simulink model "stm32g474_buck_vmc_discoverykit"  (R2022a)
settings: Solver=FixedStepAuto  StartTime=0.0  StopTime=inf  RelTol=1e-3  EnableMultiTasking=on
libraries: stm32f4xxblockslib x5, stm32g4xxblockslib x3, simulink x2, stm32blockslib x1, svdutilitieslib x1
settings Model: Creator=vchilapu  LastModifiedBy=User
settings SolverCC: MaxZcPerStep=1
settings OptimizationCC: DefaultUnderspecifiedDataType=single  EnhancedBackFolding=on  PassReuseOutputArgsAs=Individual arguments  ZeroExternalMemoryAtStartup=off  ZeroInternalMemoryAtStartup=off  MaxStackSize=64  OptimizeBlockOrder=speed  DifferentSizesBufferReuse=on  OptimizationCustomize=off  EfficientTunableParamExpr=on
settings DebuggingCC: ParameterPrecisionLossMsg=none  ParameterTunabilityLossMsg=error
settings HardwareCC: ProdBitPerPointer=32  ProdBitPerSizeT=32  ProdBitPerPtrDiffT=32  ProdLargestAtomicInteger=Long  ProdLargestAtomicFloat=Double  ProdWordSize=32  ProdLongLongMode=on  ProdHWDeviceType=ARM Compatible->ARM Cortex
settings SFSimCC: MATLABDynamicMemAlloc=off
settings RTWCC: SystemTargetFile=ert.tlc  HardwareBoard=STM32G4xx Based  TemplateMakefile=ert_default_tmf  GenerateReport=on  Toolchain=GNU Tools for ARM Embedded Processors  BuildConfiguration=Specify  IncludeHyperlinkInReport=on  GenerateTraceInfo=on
settings CodeAppCC: ForceParamTrailComments=on  IgnoreCustomStorageClasses=off  OperatorAnnotations=on  SimulinkDataObjDesc=on  SFDataObjDesc=on  InsertBlockDesc=on
settings ERTTargetCC: TargetLangStandard=C99 (ISO)  CodeReplacementLibrary=ARM Cortex-M  ExtModeTransport=3  ExtModeStaticAlloc=on  ExtModeStaticAllocSize=2048  ExtModeMexFile=ext_xcp  ExtModeIntrfLevel=Level2 - Open

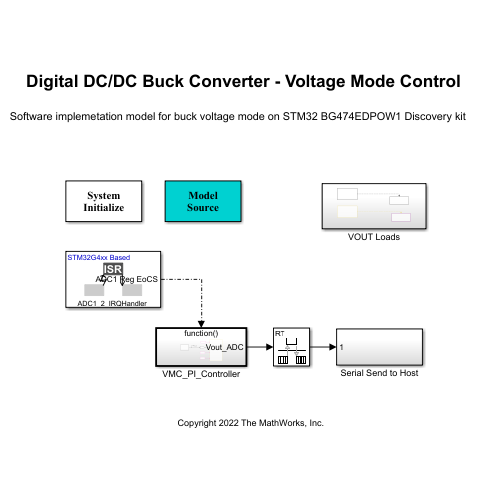
[thumbnail: Simulink's stored preview of the top-level diagram]
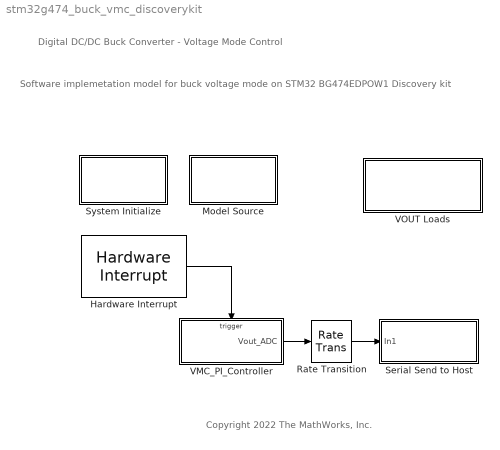
== system stm32g474_buck_vmc_discoverykit ==
  note: Digital DC/DC Buck Converter - Voltage Mode Control
  note: Software implemetation model for buck voltage mode on STM32 BG474EDPOW1 Discovery kit
  note: Copyright 2022 The MathWorks, Inc.
  Hardware Interrupt : stm32g4xxblockslib/Hardware Interrupt  ISRGroup=Analog to digital converter (ADC)  ISRName=ADC1_2_IRQHandler  ISRNumber=33  EventsList={ 'off', 'ADC1 OVR', '1'; 'on', 'ADC1 Reg EoCS', '2'; 'off', 'ADC1 Inj EoCS', '3'; 'off', 'ADC1 Inj JQOVF', '4'; 'off', 'ADC1 Watchdog1', '5'; 'off', 'ADC1 Watchdog2', '6'; 'off', 'ADC1 Watchdog3', '7'; 'off', 'ADC2 OVR', '8'; 'off', 'ADC2 Reg EoCS', '9'; 'off', 'ADC2 Inj EoCS', '10'; 'off', 'ADC2 Inj JQOVF', '11'; 'off', 'ADC2 Watchdog', '12'; 'off', 'ADC2 Watchdog2', '13'; 'off', 'ADC2 Watchdog3', '14'; 'off', 'Custom event', '15' }  SelectedEvents={'ADC1 Reg EoCS'}  TaskPriority=30  DisablePreemption=off  ClearInterruptFlagsAtEndOfEvent=off  InterruptDefinitionFile=$(TARGET_ROOT)/registry/interrupts/STM32F4xxBased_interrupts.xml  EnableSimPort=off
      settings: SourceProductBaseCode=STMICRODIS
  Model Source : Subsystem  mask(Model Source){ShowInLibBrowser=0}
      mask prompts: ShowInLibBrowser "Simulink:masks:CustCodeMaskParam1_MP"
      settings: CopyFcn=cccopyfcn(gcb)  OpenFcn=ccopenfcn('Model Source')
      mask Help: eval('feval(''rtwprivate'',''rtwhelpview'',''rtw_model_source_block'')');
      mask Display: disp('Model\nSource');
  Rate Transition : RateTransition  Integrity=off  Deterministic=off  OutPortSampleTime=20e-6
  Serial Send to Host : Subsystem
  System Initialize : Subsystem  mask(System Initialize){ShowInLibBrowser=0}
      mask prompts: ShowInLibBrowser "Simulink:masks:CustCodeMaskParam1_MP"
      settings: CopyFcn=cccopyfcn(gcb)  OpenFcn=ccopenfcn('System Initialize Function')
      mask Help: eval('feval(''rtwprivate'',''rtwhelpview'',''rtw_sys_initialize_block'')');
      mask Display: disp('System\nInitialize');
  VMC_PI_Controller : Subsystem  TreatAsAtomicUnit=on
  VOUT Loads : Subsystem
  wires:
  VMC_PI_Controller/1(Vout_ADC) -> Rate Transition/1
  Rate Transition/1 -> Serial Send to Host/1(In1)
  Hardware Interrupt/1 -> VMC_PI_Controller/Trigger

== system stm32g474_buck_vmc_discoverykit/Model Source ==

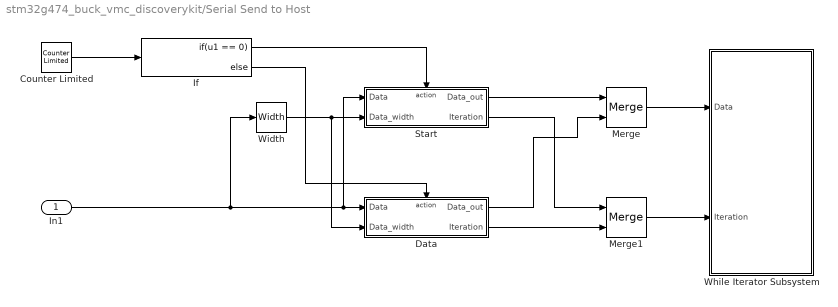
== system stm32g474_buck_vmc_discoverykit/Serial Send to Host ==
  In1 : Inport
  Counter Limited : simulink/Sources/Counter Limited  uplimit=2999  tsamp=-1
  Data : Subsystem  TreatAsAtomicUnit=on
  If : If  IfExpression=u1 == 0
  Merge : Merge
  Merge1 : Merge
  Start : Subsystem  TreatAsAtomicUnit=on
  While Iterator Subsystem : Subsystem  TreatAsAtomicUnit=on
  Width : Width  OutDataTypeMode=All ports same datatype  DataType=uint16
  wires:
  If/1 -> Start/Action
  If/2 -> Data/Action
  Counter Limited/1 -> If/1
  Start/1(Data_out) -> Merge/1
  Data/1(Data_out) -> Merge/2
  Merge/1 -> While Iterator Subsystem/1(Data)
  Merge1/1 -> While Iterator Subsystem/2(Iteration)
  Start/2(Iteration) -> Merge1/1
  Data/2(Iteration) -> Merge1/2
  Width/1 -> Data/2(Data_width), Start/2(Data_width)
  In1/1 -> Width/1, Start/1(Data), Data/1(Data)

== system stm32g474_buck_vmc_discoverykit/System Initialize ==

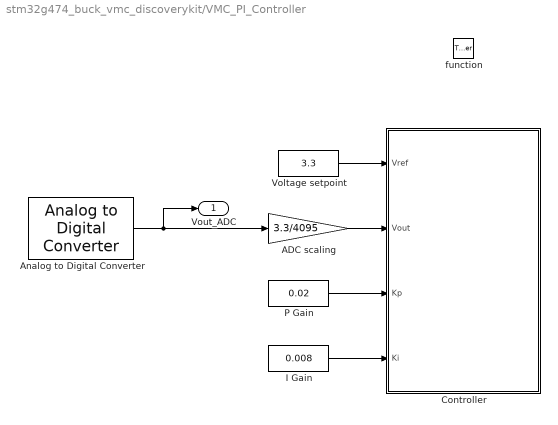
== system stm32g474_buck_vmc_discoverykit/VMC_PI_Controller ==
  function : TriggerPort  TriggerType=function-call  VariantControl=(inherit)
  ADC scaling : Gain  Gain=3.3/4095  OutDataTypeStr=single
  Analog to Digital Converter : stm32f4xxblockslib/Analog to Digital Converter  ADCModule=ADC1  ConversionGroup=Regular  TriggerMode=Read results only  NumberOfConversions=1  OutputStatus=off  SampleTime=-1  EnableSimPort=off
      settings: SourceProductBaseCode=STMICRODIS
  Controller : Subsystem
  I Gain : Constant  Value=0.008  VectorParams1D=off  OutDataTypeStr=Inherit: Inherit via back propagation
  P Gain : Constant  Value=0.02  OutDataTypeStr=Inherit: Inherit via back propagation
  Voltage setpoint : Constant  Value=3.3  OutDataTypeStr=Inherit: Inherit via back propagation
  Vout_ADC : Outport
  wires:
  ADC scaling/1 -> Controller/2(Vout)
  P Gain/1 -> Controller/3(Kp)
  I Gain/1 -> Controller/4(Ki)
  Analog to Digital Converter/1 -> Vout_ADC/1, ADC scaling/1
  Voltage setpoint/1 -> Controller/1(Vref)

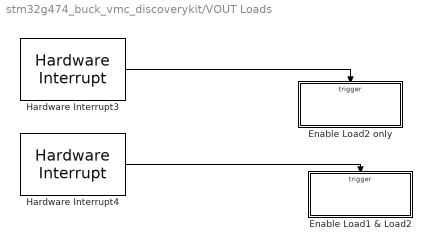
== system stm32g474_buck_vmc_discoverykit/VOUT Loads ==
  Enable Load1 & Load2 : Subsystem  TreatAsAtomicUnit=on
  Enable Load2 only : Subsystem  TreatAsAtomicUnit=on
  Hardware Interrupt3 : stm32g4xxblockslib/Hardware Interrupt  ISRGroup=External interrupts (EXTI)  ISRName=EXTI2_IRQHandler  ISRNumber=23  EventsList={ 'on', 'EXTI2 Event', '1'; 'off', 'Custom event', '2' }  SelectedEvents={'EXTI2 Event'}  TaskPriority=30  DisablePreemption=off  ClearInterruptFlagsAtEndOfEvent=off  InterruptDefinitionFile=$(TARGET_ROOT)/registry/interrupts/STM32F4xxBased_interrupts.xml  EnableSimPort=off
      settings: SourceProductBaseCode=STMICRODIS
  Hardware Interrupt4 : stm32g4xxblockslib/Hardware Interrupt  ISRGroup=External interrupts (EXTI)  ISRName=EXTI4_IRQHandler  ISRNumber=25  EventsList={ 'on', 'EXTI4 Event', '1'; 'off', 'Custom event', '2' }  SelectedEvents={'EXTI4 Event'}  TaskPriority=30  DisablePreemption=off  ClearInterruptFlagsAtEndOfEvent=off  InterruptDefinitionFile=$(TARGET_ROOT)/registry/interrupts/STM32F4xxBased_interrupts.xml  EnableSimPort=off
      settings: SourceProductBaseCode=STMICRODIS
  wires:
  Hardware Interrupt3/1 -> Enable Load2 only/Trigger
  Hardware Interrupt4/1 -> Enable Load1 & Load2/Trigger

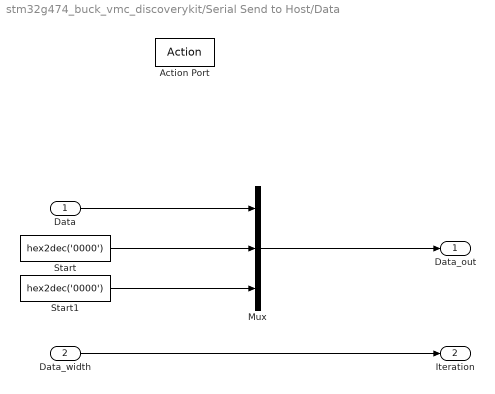
== system stm32g474_buck_vmc_discoverykit/Serial Send to Host/Data ==
  Data : Inport
  Data_width : Inport  Port=2
  Action Port : ActionPort  ActionPortLabel=else
  Mux : Mux  Inputs=3
  Start : Constant  Value=hex2dec('0000')  OutDataTypeStr=uint16
  Start1 : Constant  Value=hex2dec('0000')  OutDataTypeStr=uint16
  Data_out : Outport  VectorParamsAs1DForOutWhenUnconnected=off
  Iteration : Outport  Port=2  VectorParamsAs1DForOutWhenUnconnected=off
  wires:
  Start/1 -> Mux/2
  Mux/1 -> Data_out/1
  Data/1 -> Mux/1
  Data_width/1 -> Iteration/1
  Start1/1 -> Mux/3

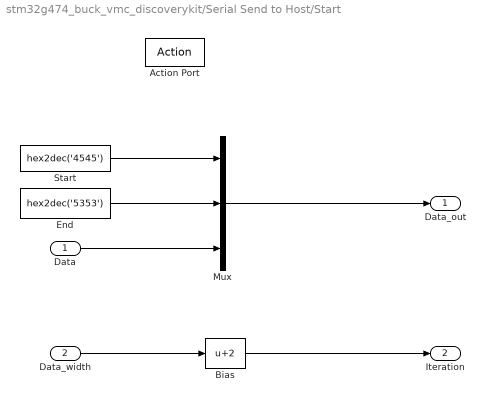
== system stm32g474_buck_vmc_discoverykit/Serial Send to Host/Start ==
  Data : Inport
  Data_width : Inport  Port=2
  Action Port : ActionPort  ActionPortLabel=if(u1 == 0)
  Bias : Bias  Bias=2  SaturateOnIntegerOverflow=off
  End : Constant  Value=hex2dec('5353')  OutDataTypeStr=uint16
  Mux : Mux  Inputs=3
  Start : Constant  Value=hex2dec('4545')  OutDataTypeStr=uint16
  Data_out : Outport  VectorParamsAs1DForOutWhenUnconnected=off
  Iteration : Outport  Port=2  VectorParamsAs1DForOutWhenUnconnected=off
  wires:
  End/1 -> Mux/2
  Mux/1 -> Data_out/1
  Data_width/1 -> Bias/1
  Bias/1 -> Iteration/1
  Data/1 -> Mux/3
  Start/1 -> Mux/1

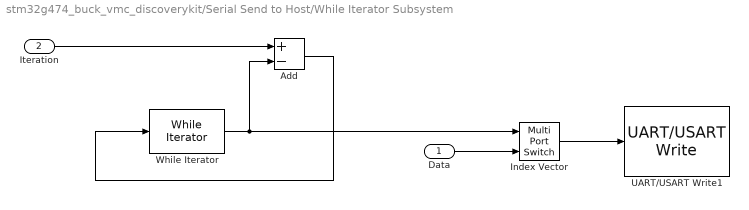
== system stm32g474_buck_vmc_discoverykit/Serial Send to Host/While Iterator Subsystem ==
  Data : Inport
  Iteration : Inport  Port=2
  Add : Sum  Inputs=+-  OutDataTypeStr=Inherit: Same as first input
  Index Vector : MultiPortSwitch  Inputs=1  SaturateOnIntegerOverflow=off  InputSameDT=off
  UART/USART Write1 : stm32blockslib/UART//USART Write  Priority=1  UARTModule=USART3  LengthOfDataToSend=off  BlockingMode=on  BlockingTimeout=1  OutputStatus=off
      settings: SourceProductBaseCode=STMICRODIS
  While Iterator : WhileIterator  MaxIters=-1  WhileBlockType=do-while  ShowIterationPort=on  OutputDataType=int16
  wires:
  Iteration/1 -> Add/1
  Add/1 -> While Iterator/1
  Index Vector/1 -> UART/USART Write1/1
  Data/1 -> Index Vector/2
  While Iterator/1 -> Index Vector/1, Add/2

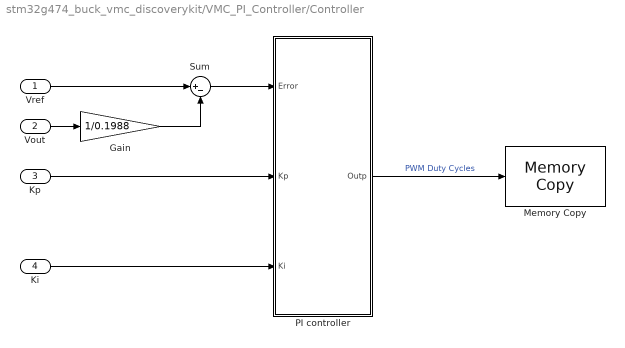
== system stm32g474_buck_vmc_discoverykit/VMC_PI_Controller/Controller ==
  Vref : Inport
  Vout : Inport  Port=2
  Kp : Inport  Port=3
  Ki : Inport  Port=4
  Gain : Gain  Gain=1/0.1988
  Memory Copy : svdutilitieslib/Memory Copy  copyFrom=Input port  copyFromAddressSource=Specify via dialog  copyFromAddress=hex2dec('00001000')  copyFromSrcCode=myVariableSrc  dataTypeFrom=Inherit from input port  dataDimensionFrom=1  useOffsetFrom=off  offsetFromSrc=Specify via dialog  offsetFrom=0  strideFrom=1  copyTo=Specified source code symbol  copyToAddressSource=Specify via dialog  copyToAddress=&HRTIMC->sTimerxRegs[3].CMP2xR  copyToSrcCode=&HRTIMC->sTimerxRegs[2].CMP1xR  dataTypeTo=uint32  useOffsetTo=off  offsetToSrc=Specify via dialog  offsetTo=0  strideTo=1  sampleTime=-1  useInitValue=off  initValueSrc=Specify constant value  initValue=1  initValueSrcCode=myInitValueVariable  useAsMask=off  maskOperator=bitwise AND  useTermValue=off  termValue=1  isRealtimeEnabled=off  emitCCBeforeWrite=off  CCBeforeWrite=/* Custom Code Before Write*/  emitCCAfterWrite=off  CCAfterWrite=/* Custom Code After Write*/  useDMACopy=off  enableBlockingMode=off  blockPlatform=stm32f4discovery
      settings: SourceProductBaseCode=ANDROID,ARDUINO,ML_ARDUINO,ECCORTEXA,ECCORTEXR,SC_BEAGLEBONE_BLUE,EC_FREEDOM_BOARD,EC_FRDM_K64F,INTEL_BLOCKSET,MICROBIT,NUCLEO,NVIDIA,PX4AUTOPILOTS,RASPPIIO,STMICRODIS,TIC2000,XILINX_BLOCKSET
  PI controller : Subsystem
  Sum : Sum  Inputs=|+-
  wires:
  Kp/1 -> PI controller/2(Kp)
  Ki/1 -> PI controller/3(Ki)
  Vref/1 -> Sum/1
  Vout/1 -> Gain/1
  Sum/1 -> PI controller/1(Error)
  Gain/1 -> Sum/2
  PI controller/1(Outp) -> Memory Copy/1  "PWM Duty Cycles"

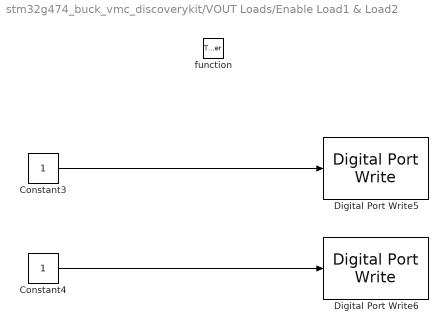
== system stm32g474_buck_vmc_discoverykit/VOUT Loads/Enable Load1 & Load2 ==
  function : TriggerPort  TriggerType=function-call  VariantControl=(inherit)
  Constant3 : Constant
  Constant4 : Constant
  Digital Port Write5 : stm32f4xxblockslib/Digital Port Write  PortName=GPIOC  PinNumber=[14]  ReadOperation=off  IOAsArray=on  EnableSimPort=off
      settings: SourceProductBaseCode=STMICRODIS
  Digital Port Write6 : stm32f4xxblockslib/Digital Port Write  PortName=GPIOC  PinNumber=[15]  ReadOperation=off  IOAsArray=on  EnableSimPort=off
      settings: SourceProductBaseCode=STMICRODIS
  wires:
  Constant3/1 -> Digital Port Write5/1
  Constant4/1 -> Digital Port Write6/1

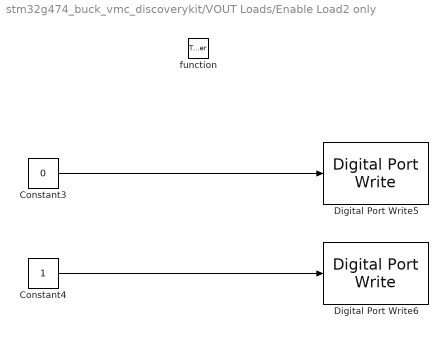
== system stm32g474_buck_vmc_discoverykit/VOUT Loads/Enable Load2 only ==
  function : TriggerPort  TriggerType=function-call  VariantControl=(inherit)
  Constant3 : Constant  Value=0
  Constant4 : Constant
  Digital Port Write5 : stm32f4xxblockslib/Digital Port Write  PortName=GPIOC  PinNumber=[14]  ReadOperation=off  IOAsArray=on  EnableSimPort=off
      settings: SourceProductBaseCode=STMICRODIS
  Digital Port Write6 : stm32f4xxblockslib/Digital Port Write  PortName=GPIOC  PinNumber=[15]  ReadOperation=off  IOAsArray=on  EnableSimPort=off
      settings: SourceProductBaseCode=STMICRODIS
  wires:
  Constant3/1 -> Digital Port Write5/1
  Constant4/1 -> Digital Port Write6/1

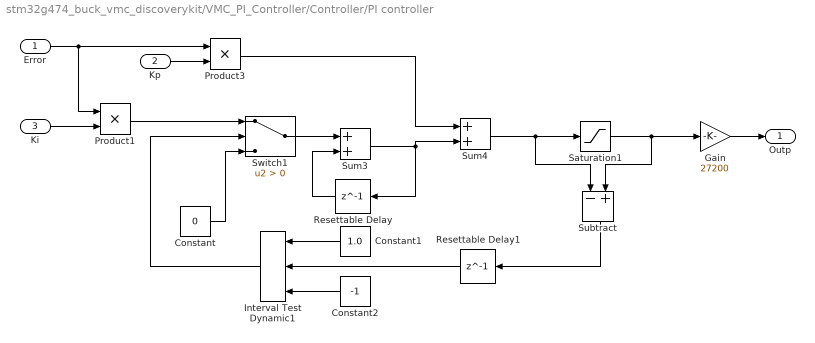
== system stm32g474_buck_vmc_discoverykit/VMC_PI_Controller/Controller/PI controller ==
  Error : Inport
  Kp : Inport  Port=2
  Ki : Inport  Port=3
  Constant : Constant  Value=0  OutDataTypeStr=Inherit: Inherit via back propagation
  Constant1 : Constant  Value=1.0  OutDataTypeStr=Inherit: Inherit via back propagation
  Constant2 : Constant  Value=-1  OutDataTypeStr=Inherit: Inherit via back propagation
  Gain : Gain  Gain=27200  ParamDataTypeStr=uint16  OutDataTypeStr=uint16
  Interval Test Dynamic1 : simulink/Logic and Bit Operations/Interval Test Dynamic  IntervalClosedRight=on  IntervalClosedLeft=on  OutDataTypeStr=boolean
      settings: SourceProductBaseCode=SL
  Product1 : Product
  Product3 : Product
  Resettable Delay : Delay  DelayLength=1
  Resettable Delay1 : Delay  DelayLength=1
  Saturation1 : Saturate  UpperLimit=0.8  LowerLimit=0.0  LinearizeAsGain=off
  Subtract : Sum  Inputs=-+
  Sum3 : Sum
  Sum4 : Sum
  Switch1 : Switch  Criteria=u2 > Threshold  SaturateOnIntegerOverflow=off  InputSameDT=off
  Outp : Outport  VectorParamsAs1DForOutWhenUnconnected=off
  wires:
  Resettable Delay1/1 -> Interval Test Dynamic1/2
  Gain/1 -> Outp/1
  Constant2/1 -> Interval Test Dynamic1/3
  Interval Test Dynamic1/1 -> Switch1/2
  Subtract/1 -> Resettable Delay1/1
  Switch1/1 -> Sum3/1
  Ki/1 -> Product1/2
  Sum4/1 -> Saturation1/1, Subtract/1
  Product3/1 -> Sum4/1
  Product1/1 -> Switch1/1
  Sum3/1 -> Sum4/2, Resettable Delay/1
  Error/1 -> Product1/1, Product3/1
  Kp/1 -> Product3/2
  Resettable Delay/1 -> Sum3/2
  Constant/1 -> Switch1/3
  Constant1/1 -> Interval Test Dynamic1/1
  Saturation1/1 -> Subtract/2, Gain/1
